simulink model "pidinputquaternion"  (R2014a)
settings: Solver=ode45  StartTime=0.0  StopTime=10  RelTol=1e-3
libraries: aerolibutil x2, dspinverses x1
settings Model: Creator=aman  LastModifiedBy=aman

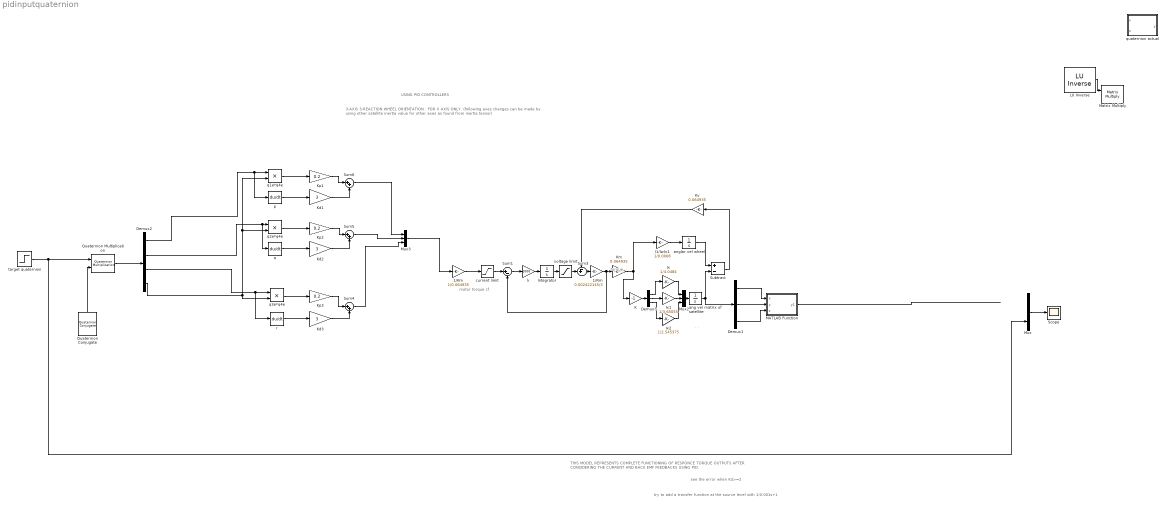
== system pidinputquaternion ==
  note: .
      |
      | .
  note: try to add a transfer function at the source level with 1/0.001s+1
  note: see the error when Kd>=2
  note: USING PID CONTROLLERS
  note: 3-AXIS 3-REACTION WHEEL ORIENTATION : FOR X AXIS ONLY.
      | (following axes changes can be made by using other satellite inertia value for other axes as found from inertia tensor)
  note: torque
  note: THIS MODEL REPRESENTS COMPLETE FUNCTIONING OF RESPONCE TORQUE OUTPUTS AFTER CONSIDERING THE CURRENT AND BACK EMF FEEDBACKS USING PID.
  note: motor
      | torque
      | cf.
  " LU Inverse" : dspinverses/ LU Inverse
  (1/Iw)x1 : Gain  Gain=1/0.0008
  1/Km : Gain  Gain=1/0.064935
  1/Rm : Gain  Gain=0.002422145/3
  Demux1 : Demux  Outputs=3
  Demux2 : Demux
  Demux3 : Demux  Outputs=3
  Integrator : Integrator
  Ix : Gain  Gain=1/4.0484
  Ix1 : Gain  Gain=1/3.65055
  Ix2 : Gain  Gain=1/2.545375
  K : Gain  Gain=-1
  Kd1 : Gain  Gain=3
  Kd2 : Gain  Gain=3
  Kd3 : Gain  Gain=3
  Km : Gain  Gain=0.064935
  Kp1 : Gain  Gain=0.2
  Kp2 : Gain  Gain=0.2
  Kp3 : Gain  Gain=0.2
  Kv : Gain  Gain=0.064935
  MATLAB Function : MATLAB Function  TreatAsAtomicUnit=on
  Matrix Multiply : Product  Multiplication=Matrix(*)
  Mux : Mux  Inputs=2
  Mux2 : Mux  Inputs=3
  Mux3 : Mux  Inputs=3
  Quaternion Conjugate : aerolibutil/Quaternion Conjugate
  Quaternion Multiplication : aerolibutil/Quaternion Multiplication
  Scope : Scope
      settings: SaveName=ScopeData2
  Subtract : Sum  Inputs=+-
  Sum1 : Sum  Inputs=|+-
  Sum3 : Sum  Inputs=-+|
  Sum4 : Sum  Inputs=|++
  Sum5 : Sum  Inputs=|++
  Sum6 : Sum  Inputs=|++
  ang vel matrix of satellite : Integrator
  anglar vel wheel : Integrator
  current limit : Saturate  UpperLimit=0.0816  LowerLimit=-0.016
  k : Gain  Gain=1000
  p : Derivative
  q : Derivative
  q1e*q4e : Product
  q2e*q4e : Product
  q3e*q4e : Product
  quaternion actual : MATLAB Function  TreatAsAtomicUnit=on
  r : Derivative
  target quaternion : Step  Before=[0;0;0;0]  After=[4;5;3;0]  SampleTime=0
  voltage limit : Saturate  UpperLimit=34  LowerLimit=-34
  wires:
  1/Km/1 -> current limit/1
  k/1 -> Integrator/1
  Integrator/1 -> voltage limit/1
  1/Rm/1 -> Sum1/2, Km/1
  current limit/1 -> Sum1/1
  Sum1/1 -> k/1
  Sum3/1 -> 1/Rm/1
  voltage limit/1 -> Sum3/2
  Mux3/1 -> 1/Km/1
  Demux2/4 -> q3e*q4e/2, q1e*q4e/2, q2e*q4e/2
  q1e*q4e/1 -> Kp1/1
  q2e*q4e/1 -> Kp2/1
  q3e*q4e/1 -> Kp3/1
  p/1 -> Kd1/1
  q/1 -> Kd2/1
  r/1 -> Kd3/1
  Kp1/1 -> Sum6/1
  Kd1/1 -> Sum6/2
  Kp2/1 -> Sum5/1
  Kd2/1 -> Sum5/2
  Kp3/1 -> Sum4/1
  Kd3/1 -> Sum4/2
  Sum6/1 -> Mux3/1
  Sum5/1 -> Mux3/2
  Sum4/1 -> Mux3/3
  Km/1 -> K/1, (1/Iw)x1/1
  (1/Iw)x1/1 -> anglar vel wheel/1
  anglar vel wheel/1 -> Subtract/1
  Subtract/1 -> Kv/1
  Kv/1 -> Sum3/1
  Demux2/3 -> r/1, q3e*q4e/1
  Demux2/2 -> q/1, q2e*q4e/1
  Demux2/1 -> q1e*q4e/1, p/1
  Mux/1 -> Scope/1
  target quaternion/1 -> Quaternion Multiplication/1, Mux/2
  ? -> Quaternion Conjugate/1
  Quaternion Conjugate/1 -> Quaternion Multiplication/2
  " LU Inverse"/1 -> Matrix Multiply/1
  ang vel matrix of satellite/1 -> Subtract/2, Demux1/1
  Quaternion Multiplication/1 -> Demux2/1
  Demux3/2 -> Ix1/1
  Demux3/3 -> Ix2/1
  Demux3/1 -> Ix/1
  Mux2/1 -> ang vel matrix of satellite/1
  Ix/1 -> Mux2/1
  Ix1/1 -> Mux2/2
  Ix2/1 -> Mux2/3
  ? -> Matrix Multiply/2
  Demux1/1 -> MATLAB Function/1(x)
  Demux1/2 -> MATLAB Function/2(y)
  Demux1/3 -> MATLAB Function/3(z)
  K/1 -> Demux3/1
  MATLAB Function/1(y1) -> ?

== matlab function pidinputquaternion/MATLAB Function ==
  data: x input; y input; z input; y1 output
function y1 = fcn(x, y, z)
%#codegen

y1 = [0 z -y x; -z 0 x y; y -x 0 z; -x -y -z 0];

== matlab function pidinputquaternion/quaternion actual ==
  data: v input; u input; y output
function y = fcn(v,u)
%#codegen

y = 2*(v/u);
